simulink model "DesEn"  (Simulink 7.5)
settings: Solver=ode45  StartTime=0.0  StopTime=10  RelTol=1e-3
values from neighbouring files (symbols this model uses):
  Key = u2'    [Input.m]
  P = [16,7,20,21,29,12,28,17,1,15,23,26,5,18,31,10,2,8,24,14,32,27,3,9,19,13,30,6,22,11,4,25]    [Des.m]    (also in Input.m = u1')
settings Model: Creator=jixuebin  LastModifiedBy=jixuebin

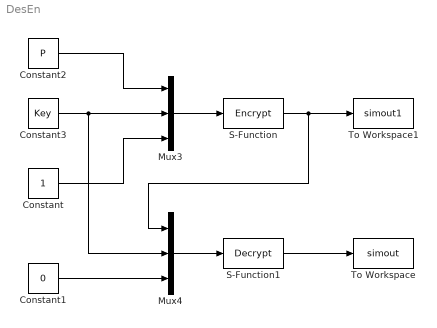
== system DesEn ==
  Constant : Constant  OutDataType=fixdt(1, 16)  OutScaling=2^0
  Constant1 : Constant  Value=0  OutDataType=fixdt(1, 16)  OutScaling=2^0
  Constant2 : Constant  Value=P  OutDataType=fixdt(1, 16)  OutScaling=2^0
  Constant3 : Constant  Value=Key  OutDataType=fixdt(1, 16)  OutScaling=2^0
  Mux3 : Mux  Inputs=3
  Mux4 : Mux  Inputs=3
  S-Function : S-Function  FunctionName=Encrypt  EnableBusSupport=off
  S-Function1 : S-Function  FunctionName=Decrypt  EnableBusSupport=off
  To Workspace : ToWorkspace  VariableName=simout  SampleTime=-1  SaveFormat=Structure
  To Workspace1 : ToWorkspace  VariableName=simout1  SampleTime=-1  SaveFormat=Structure
  wires:
  Constant3/1 -> Mux3/2, Mux4/2
  Constant/1 -> Mux3/3
  Constant2/1 -> Mux3/1
  Mux3/1 -> S-Function/1
  Constant1/1 -> Mux4/3
  S-Function1/1 -> To Workspace/1
  Mux4/1 -> S-Function1/1
  S-Function/1 -> Mux4/1, To Workspace1/1
